simulink model "CruiseControl_VS_harness"  (R2015b)
settings: Solver=FixedStepDiscrete  StartTime=0.0  StopTime=Inf  FixedStep=0.1  RelTol=1e-3
model workspace (MAT data in the model file):
  AccelResSw = mpt.Signal
  AccelResSw.DataType = 'boolean'
  AccelResSw.Min = 0
  AccelResSw.Max = 1
  AccelResSw.Dimensions = 1
  AccelResSw.DimensionsMode = 'Fixed'
  AccelResSw.Complexity = 'auto'
  AccelResSw.SampleTime = -1
  AccelResSw.SamplingMode = 'auto'
  Brake = mpt.Signal
  Brake.DataType = 'boolean'
  Brake.Min = 0
  Brake.Max = 1
  Brake.Dimensions = 1
  Brake.DimensionsMode = 'Fixed'
  Brake.Complexity = 'auto'
  Brake.SampleTime = -1
  Brake.SamplingMode = 'auto'
  CoastSetSw = mpt.Signal
  CoastSetSw.DataType = 'boolean'
  CoastSetSw.Min = 0
  CoastSetSw.Max = 1
  CoastSetSw.Dimensions = 1
  CoastSetSw.DimensionsMode = 'Fixed'
  CoastSetSw.Complexity = 'auto'
  CoastSetSw.SampleTime = -1
  CoastSetSw.SamplingMode = 'auto'
  CruiseOnOff = mpt.Signal
  CruiseOnOff.DataType = 'boolean'
  CruiseOnOff.Min = 0
  CruiseOnOff.Max = 1
  CruiseOnOff.Dimensions = 1
  CruiseOnOff.DimensionsMode = 'Fixed'
  CruiseOnOff.Complexity = 'auto'
  CruiseOnOff.SampleTime = -1
  CruiseOnOff.SamplingMode = 'auto'
  Speed = mpt.Signal
  Speed.DataType = 'uint8'
  Speed.Min = 0
  Speed.Max = 160
  Speed.Dimensions = 1
  Speed.DimensionsMode = 'Fixed'
  Speed.Complexity = 'auto'
  Speed.SampleTime = -1
  Speed.SamplingMode = 'auto'
  engaged = mpt.Signal
  engaged.DataType = 'boolean'
  engaged.Min = 0
  engaged.Max = 1
  engaged.Dimensions = 1
  engaged.DimensionsMode = 'Fixed'
  engaged.Complexity = 'auto'
  engaged.SampleTime = -1
  engaged.SamplingMode = 'auto'
  holdrate = mpt.Parameter
  holdrate.Value = 5
  holdrate.DataType = 'uint8'
  holdrate.Min = 1
  holdrate.Max = 10
  incdec = mpt.Parameter
  incdec.Value = 1
  incdec.DataType = 'uint8'
  incdec.Min = 1
  incdec.Max = 2
  maxtspeed = mpt.Parameter
  maxtspeed.Value = 90
  maxtspeed.DataType = 'uint8'
  maxtspeed.Min = 80
  maxtspeed.Max = 90
  mintspeed = mpt.Parameter
  mintspeed.Value = 20
  mintspeed.DataType = 'uint8'
  mintspeed.Min = 20
  mintspeed.Max = 25
  tspeed = mpt.Signal
  tspeed.DataType = 'uint8'
  tspeed.Min = 0
  tspeed.Max = 160
  tspeed.Dimensions = 1
  tspeed.DimensionsMode = 'Fixed'
  tspeed.Complexity = 'auto'
  tspeed.SampleTime = -1
  tspeed.SamplingMode = 'auto'
libraries: aerolibanimutils x1
settings Model: PauseTimes=1.5  Creator=colosky  LastModifiedBy=colosky
settings DataIOCC: LimitDataPoints=off  SaveFormat=Array  SaveOutput=off  InspectSignalLogs=on  SaveTime=off
settings OptimizationCC: OptimizeModelRefInitCode=on  LifeSpan=Inf
settings DebuggingCC: UnderspecifiedInitializationDetection=Classic  MergeDetectMultiDrivingBlocksExec=none  SolverPrmCheckMsg=warning
settings HardwareCC: ProdBitPerPointer=32  ProdLargestAtomicFloat=None  ProdIntDivRoundTo=Undefined  ProdEndianess=Unspecified  ProdWordSize=32  ProdHWDeviceType=32-bit Generic
settings RTWCC: SystemTargetFile=ert.tlc  TemplateMakefile=ert_default_tmf  Description=Embedded Coder  SILDebugging=on
settings CodeAppCC: IgnoreCustomStorageClasses=off
settings ERTTargetCC: GenerateSampleERTMain=on  ERTCustomFileTemplate=example_file_process.tlc
settings ConfigComp: CovMetricSettings=dcmw  CovHTMLOptions=-sRT=1 -sVT=0 -aTS=0 -bRG=1 -bTC=1 -hTR=0 -nFC=0 -scm=1 -bcm=1 -xEv=0  CovSaveSingleToWorkspaceVar=off  CovCumulativeReport=on  CovReportOnPause=off  CovModelRefEnable=all  CovSFcnEnable=off

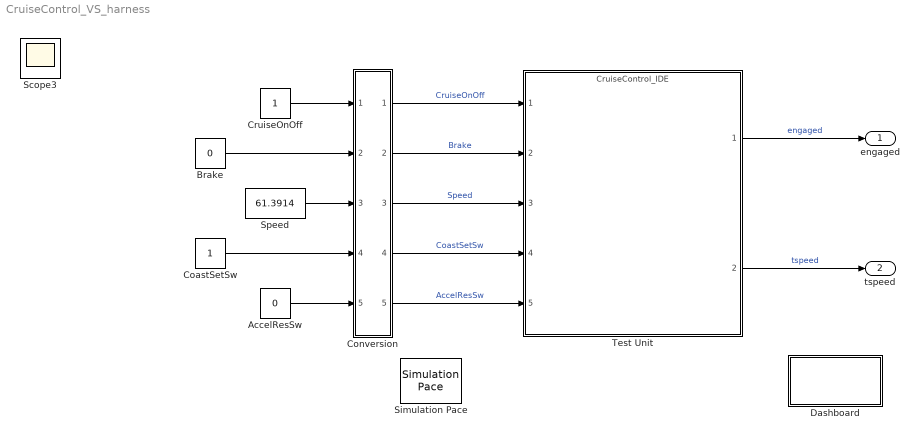
== system CruiseControl_VS_harness ==
  AccelResSw : Constant  Value=0  OutDataTypeStr=boolean
      settings: OpenFcn=|
      | val = ~str2num(get_param(gcb,'Value'));
      | set_param(gcb,'Value',num2str(val));
      | if val
      |    set_param(gcb,'BackgroundColor','green');
      | else
      |    set_param(gcb,'BackgroundColor','red');
      | end
  Brake : Constant  Value=0  OutDataTypeStr=boolean
      settings: OpenFcn=|
      | val = ~str2num(get_param(gcb,'Value'));
      | set_param(gcb,'Value',num2str(val));
      | if val
      |    set_param(gcb,'BackgroundColor','green');
      | else
      |    set_param(gcb,'BackgroundColor','red');
      | end
  CoastSetSw : Constant  OutDataTypeStr=boolean
      settings: OpenFcn=|
      | val = ~str2num(get_param(gcb,'Value'));
      | set_param(gcb,'Value',num2str(val));
      | if val
      |    set_param(gcb,'BackgroundColor','green');
      | else
      |    set_param(gcb,'BackgroundColor','red');
      | end
  Conversion : Subsystem
      mask Display: disp(['Data' char(10) 'Type' char(10) 'Conv']);
  CruiseOnOff : Constant  OutDataTypeStr=boolean
      settings: OpenFcn=|
      | val = ~str2num(get_param(gcb,'Value'));
      | set_param(gcb,'Value',num2str(val));
      | if val
      |    set_param(gcb,'BackgroundColor','green');
      | else
      |    set_param(gcb,'BackgroundColor','red');
      | end
  Dashboard : Subsystem
      mask Display: disp('Dashboard');
  Simulation Pace : aerolibanimutils/Simulation Pace  SimulationPace=1  SleepMode=MATLAB Thread  OutputPaceError=off  SampleTime=-1
      settings: AttributesFormatString=%<SimulationPace> sec/sec
  Speed : Constant  Value=61.3914  OutMin=0  OutMax=120  OutDataTypeStr=Inherit: Inherit via back propagation
  Test Unit : ModelReference  ModelNameDialog=CruiseControl_IDE  SimulationMode=Software-in-the-loop (SIL)  CodeInterface=Top model  ModelReferenceVersion=1.458  CopyOfModelName=CruiseControl_IDE
  engaged : Outport
  tspeed : Outport  Port=2
  Scope3 : Scope
  wires:
  Conversion/1(Out1) -> Test Unit/1  "CruiseOnOff"
  Conversion/5(Out5) -> Test Unit/5  "AccelResSw"
  Conversion/2(Out2) -> Test Unit/2  "Brake"
  Conversion/4(Out4) -> Test Unit/4  "CoastSetSw"
  Conversion/3(Out3) -> Test Unit/3  "Speed"
  CruiseOnOff/1 -> Conversion/1(In1)
  Brake/1 -> Conversion/2(In2)
  Speed/1 -> Conversion/3(In3)
  CoastSetSw/1 -> Conversion/4(In4)
  AccelResSw/1 -> Conversion/5(In5)
  Test Unit/1 -> engaged/1  "engaged"
  Test Unit/2 -> tspeed/1  "tspeed"

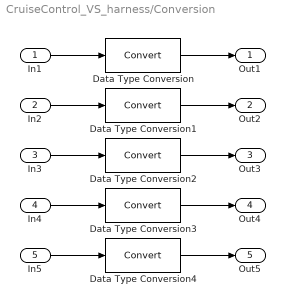
== system CruiseControl_VS_harness/Conversion ==
  In1 : Inport
  In2 : Inport  Port=2
  In3 : Inport  Port=3
  In4 : Inport  Port=4
  In5 : Inport  Port=5
  Data Type Conversion{,1..4} (5 alike) : DataTypeConversion
  Out1 : Outport
  Out2 : Outport  Port=2
  Out3 : Outport  Port=3
  Out4 : Outport  Port=4
  Out5 : Outport  Port=5
  wires:
  In4/1 -> Data Type Conversion3/1
  Data Type Conversion4/1 -> Out5/1
  Data Type Conversion1/1 -> Out2/1
  In1/1 -> Data Type Conversion/1
  Data Type Conversion/1 -> Out1/1
  In5/1 -> Data Type Conversion4/1
  In2/1 -> Data Type Conversion1/1
  Data Type Conversion3/1 -> Out4/1
  In3/1 -> Data Type Conversion2/1
  Data Type Conversion2/1 -> Out3/1

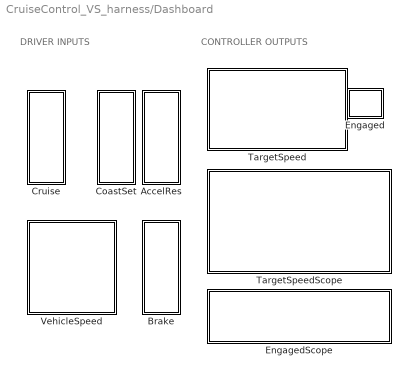
== system CruiseControl_VS_harness/Dashboard ==
  note: CONTROLLER OUTPUTS
  note: DRIVER INPUTS
  AccelRes : Subsystem  DialogController=hmiCreateDDGDialog  IsWebBlock=on  mask(MathWorksWebBlock){webBlockId=bbd5d4ff-1920-46bf-8388-7b89b1be1edf, webBlockType=rockerswitch, ShowInLibBrowser=on, ShowInitialText=on, HMISrcModelName=CruiseControl_IDE_harness}
      mask prompts: webBlockId "WebBlock Id"; webBlockType "WebBlock Type"; HMISrcModelName "Source Model"
      mask Help: helpview([docroot '/mapfiles/simulink.map'], 'hmi_rocker_switch')
      mask Display:
      | if strcmp(get_param(bdroot(gcb),'BlockDiagramType'), 'library')
      |     image([(matlabroot) '/toolbox/simulink/hmi/icons/RockerSwitch.png']);
      | end
  Brake : Subsystem  DialogController=hmiCreateDDGDialog  IsWebBlock=on  mask(MathWorksWebBlock){webBlockId=559b308e-b7f8-4e26-b519-2a28583e2c0b, webBlockType=rockerswitch, ShowInLibBrowser=on, ShowInitialText=on, HMISrcModelName=CruiseControl_IDE_harness}
      mask prompts: webBlockId "WebBlock Id"; webBlockType "WebBlock Type"; HMISrcModelName "Source Model"
      mask Help: helpview([docroot '/mapfiles/simulink.map'], 'hmi_rocker_switch')
      mask Display:
      | if strcmp(get_param(bdroot(gcb),'BlockDiagramType'), 'library')
      |     image([(matlabroot) '/toolbox/simulink/hmi/icons/RockerSwitch.png']);
      | end
  CoastSet : Subsystem  DialogController=hmiCreateDDGDialog  IsWebBlock=on  mask(MathWorksWebBlock){webBlockId=64c7b100-e804-4953-b991-e5daffb12d78, webBlockType=rockerswitch, ShowInLibBrowser=on, ShowInitialText=on, HMISrcModelName=CruiseControl_IDE_harness}
      mask prompts: webBlockId "WebBlock Id"; webBlockType "WebBlock Type"; HMISrcModelName "Source Model"
      mask Help: helpview([docroot '/mapfiles/simulink.map'], 'hmi_rocker_switch')
      mask Display:
      | if strcmp(get_param(bdroot(gcb),'BlockDiagramType'), 'library')
      |     image([(matlabroot) '/toolbox/simulink/hmi/icons/RockerSwitch.png']);
      | end
  Cruise : Subsystem  DialogController=hmiCreateDDGDialog  IsWebBlock=on  mask(MathWorksWebBlock){webBlockId=4f6240e9-6de7-44f6-bbb2-bca7edce96d5, webBlockType=rockerswitch, ShowInLibBrowser=on, ShowInitialText=on, HMISrcModelName=CruiseControl_IDE_harness}
      mask prompts: webBlockId "WebBlock Id"; webBlockType "WebBlock Type"; HMISrcModelName "Source Model"
      mask Help: helpview([docroot '/mapfiles/simulink.map'], 'hmi_rocker_switch')
      mask Display:
      | if strcmp(get_param(bdroot(gcb),'BlockDiagramType'), 'library')
      |     image([(matlabroot) '/toolbox/simulink/hmi/icons/RockerSwitch.png']);
      | end
  Engaged : Subsystem  DialogController=hmiCreateDDGDialog  IsWebBlock=on  mask(MathWorksWebBlock){webBlockId=22250467-c307-43fa-be32-b3d0891c62ca, webBlockType=lamp, ShowInLibBrowser=on, ShowInitialText=on, HMISrcModelName=CruiseControl_IDE_harness}
      mask prompts: webBlockType "WebBlock Type"; HMISrcModelName "Source Model"
      mask Help: helpview([docroot '/mapfiles/simulink.map'], 'hmi_lamp')
      mask Display:
      | if strcmp(get_param(bdroot(gcb),'BlockDiagramType'), 'library')
      |     image([(matlabroot) '/toolbox/simulink/hmi/icons/Lamp.png']);
      | end
  EngagedScope : Subsystem  DialogController=hmiCreateDDGDialog  IsWebBlock=on  mask(MathWorksWebBlock){webBlockId=3cad4c65-803a-4caf-94c9-7521c895671d, webBlockType=sdiscope, ShowInitialText=on, HMISrcModelName=CruiseControl_IDE_harness}
      mask prompts: webBlockId "WebBlock Id"; webBlockType "WebBlock Type"; HMISrcModelName "Source Model"
      mask Help: helpview([docroot '/mapfiles/simulink.map'], 'hmi_scope')
      mask Display:
      | if strcmp(get_param(bdroot(gcb),'BlockDiagramType'), 'library')
      |     image([(matlabroot) '/toolbox/simulink/hmi/icons/DashboardScope.png']);
      | end
  TargetSpeed : Subsystem  DialogController=hmiCreateDDGDialog  IsWebBlock=on  mask(MathWorksWebBlock){webBlockId=569f913c-9cd3-4d67-af94-21fda8fb0f4d, webBlockType=semicirculargauge, ShowInLibBrowser=on, ShowInitialText=on, HMISrcModelName=CruiseControl_IDE_harness}
      mask prompts: webBlockId "WebBlock Id"; webBlockType "WebBlock Type"; HMISrcModelName "Source Model"
      mask Help: helpview([docroot '/mapfiles/simulink.map'], 'hmi_half_gauge')
      mask Display:
      | if strcmp(get_param(bdroot(gcb),'BlockDiagramType'), 'library')
      |     image([(matlabroot) '/toolbox/simulink/hmi/icons/SemicircularGauge.png']);
      | end
  TargetSpeedScope : Subsystem  DialogController=hmiCreateDDGDialog  IsWebBlock=on  mask(MathWorksWebBlock){webBlockId=eca2468c-6fba-419e-b47a-f3b69d3138b1, webBlockType=sdiscope, ShowInitialText=on, HMISrcModelName=CruiseControl_IDE_harness}
      mask prompts: webBlockId "WebBlock Id"; webBlockType "WebBlock Type"; HMISrcModelName "Source Model"
      mask Help: helpview([docroot '/mapfiles/simulink.map'], 'hmi_scope')
      mask Display:
      | if strcmp(get_param(bdroot(gcb),'BlockDiagramType'), 'library')
      |     image([(matlabroot) '/toolbox/simulink/hmi/icons/DashboardScope.png']);
      | end
  VehicleSpeed : Subsystem  DialogController=hmiCreateDDGDialog  IsWebBlock=on  mask(MathWorksWebBlock){webBlockId=e9f00648-b2c0-4db1-939b-f83e1fa6bec6, webBlockType=continuousknob, ShowInLibBrowser=on, ShowInitialText=on, HMISrcModelName=CruiseControl_IDE_harness}
      mask prompts: webBlockId "WebBlock Id"; webBlockType "WebBlock Type"; HMISrcModelName "Source Model"
      mask Help: helpview([docroot '/mapfiles/simulink.map'], 'hmi_knob')
      mask Display:
      | if strcmp(get_param(bdroot(gcb),'BlockDiagramType'), 'library')
      |     image([(matlabroot) '/toolbox/simulink/hmi/icons/ContinuousKnob.png']);
      | end

== system CruiseControl_VS_harness/Dashboard/AccelRes ==

== system CruiseControl_VS_harness/Dashboard/Brake ==

== system CruiseControl_VS_harness/Dashboard/CoastSet ==

== system CruiseControl_VS_harness/Dashboard/Cruise ==

== system CruiseControl_VS_harness/Dashboard/Engaged ==

== system CruiseControl_VS_harness/Dashboard/EngagedScope ==

== system CruiseControl_VS_harness/Dashboard/TargetSpeed ==

== system CruiseControl_VS_harness/Dashboard/TargetSpeedScope ==

== system CruiseControl_VS_harness/Dashboard/VehicleSpeed ==
